simulink model "untitled"  (R2020b)
settings: Solver=VariableStepAuto  StartTime=0.0  StopTime=10.0  RelTol=1e-3
settings Model: Creator=GoniR  LastModifiedBy=GoniR

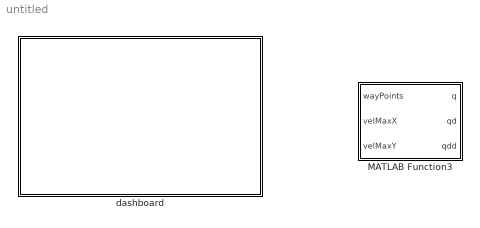
== system untitled ==
  MATLAB Function3 : MATLAB Function  TreatAsAtomicUnit=on
  dashboard : Subsystem

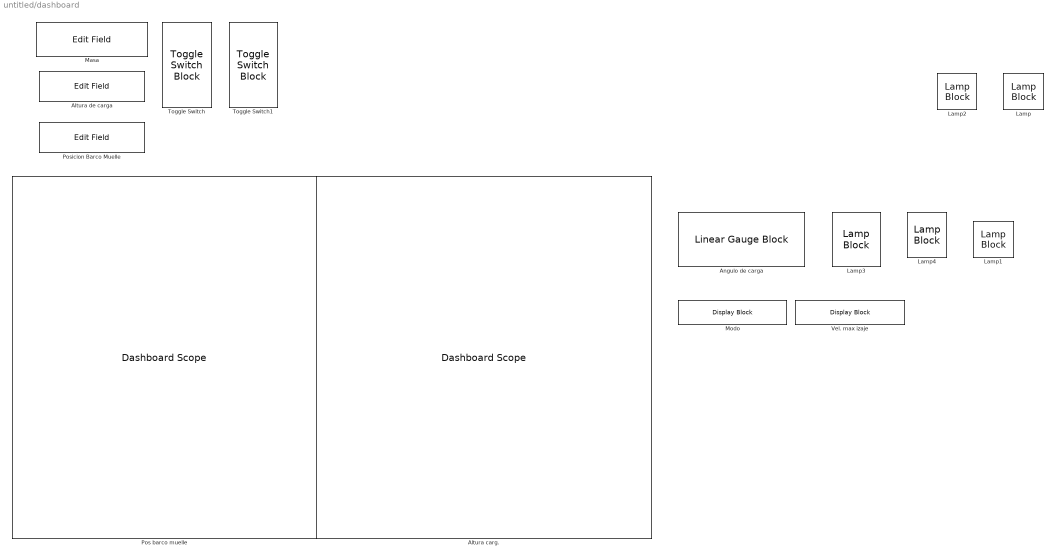
== system untitled/dashboard ==
  Altura carg. : DashboardScope
  Altura de carga : EditField  LabelPosition=Hide  ShowInitialText=on  Alignment=Center
  Angulo de carga : LinearGaugeBlock  LabelPosition=Hide  ScaleMin=-0.15  ScaleMax=0.15
  Lamp{,1..2,4} (4 alike) : LampBlock
  Lamp3 : LampBlock  LabelPosition=Bottom
  Masa : EditField  LabelPosition=Hide  ShowInitialText=on  Alignment=Center
  Modo : DisplayBlock  LabelPosition=Hide  Format=short  Transparency=1
  Pos barco muelle : DashboardScope
  Posicion Barco Muelle : EditField  LabelPosition=Hide  ShowInitialText=on  Alignment=Center
  Toggle Switch : ToggleSwitchBlock
      settings: Values={{'Off', 'On'}, [0 1]}
  Toggle Switch1 : ToggleSwitchBlock
      settings: Values={{'Sin Cambiar', 'Cambiada'}, [0 1]}
  Vel. max izaje : DisplayBlock  LabelPosition=Hide  Format=short  Transparency=1

== matlab function untitled/MATLAB Function3 ==
  data: wayPoints input size=2,100; q output size=[2,1000000]; qd output size=[2,1000000]; qdd output size=[2,1000000]; velMaxX input; velMaxY input
function [q,qd,qdd] = fcn(wayPoints,velMaxX,velMaxY)
coder.extrinsic('plot')
pendiente_ant=0;

cont_p=1;
wayPoints=wayPoints([2,1],:);
wayPoints=flip(wayPoints,2);
wayPoints(2,:)=(wayPoints(2,:)-65)*-1;
for i=1:length(wayPoints)-1
    pendiente=(wayPoints(2,i)-wayPoints(2,i+1))/(wayPoints(1,i)-wayPoints(1,i+1));
    if pendiente_ant~=pendiente
        cont_p=cont_p+1%+2;
    end
    pendiente_ant=pendiente;
end
wayPoints1=zeros(2,cont_p);
cont_p2=0;
for i=1:length(wayPoints)-1
    pendiente=(wayPoints(2,i)-wayPoints(2,i+1))/(wayPoints(1,i)-wayPoints(1,i+1));
    if pendiente_ant~=pendiente
    cont_p2=cont_p2+1%+2;
    wayPoints1(:,cont_p2)=wayPoints(:,i);
    %wayPoints1(:,cont_p2-1)=wayPoints(:,i);
    end
    pendiente_ant=pendiente;
end
wayPoints1(:,end)=wayPoints(:,end);
figure(10)
plot(wayPoints1(1,:),wayPoints1(2,:))   

vx_max=velMaxX;
vy_max=velMaxY;
vel_max=zeros(2,length(wayPoints1))


timePoints1=zeros(1,length(wayPoints1));
tiempo_ant=0;
for i=1:length(wayPoints1)-1
    restaX=abs(wayPoints1(1,i+1)-wayPoints1(1,i));
    restaY=abs(wayPoints1(2,i+1)-wayPoints1(2,i));
    timex=restaX/(vx_max/2.5);
    timey=restaY/(vy_max/2.5);
    if timex>timey
    timePoints1(i+1)=restaX/(vx_max/4)+tiempo_ant;
    elseif timex<timey
    timePoints1(i+1)=restaY/(vy_max/4)+tiempo_ant;
    else
     timePoints1(i+1)=restaX/(vx_max/4)+tiempo_ant;    
    end
    
    tiempo_ant=timePoints1(i+1);
end

tSamples1=0:1e-2:timePoints1(end);
[q,qd,qdd] = quinticpolytraj(wayPoints1,timePoints1,tSamples1)%'VelocityBoundaryCondition',vel_max);
% [q1,qd1,qdd1] = cubicpolytraj(wayPoints1,timePoints1,tSamples1);
qx=interp1(timePoints1,wayPoints1(1,:),tSamples1,'pchip');
%qx=bspline(wayPoints1(1,:));
qy=interp1(timePoints1,wayPoints1(2,:),tSamples1,'cubic');
q(1,:)=qx;
q(2,:)=qy;
figure(15)
plot(qx,qy) 
%figure(45)
%plot(tSamples1,qx) 
%figure(3)
%plot(tSamples1,qd(1,:)) 
%figure(4)
%plot(tSamples1,qdd(1,:)) 
%figure(5)
%plot(tSamples1,qdd(2,:)) 

end
